simulink model "bh_2dof_RC_orientation"  (R2016a)
settings: Solver=VariableStepAuto  StartTime=0.0  StopTime=20  RelTol=1e-3
libraries: fl_lib x26, nesl_utility x10
settings Model: Creator=bhorton  LastModifiedBy=bhorton
settings DataIOCC: LimitDataPoints=on
settings DebuggingCC: AllowSymbolicDim=off
settings ModelReferenceCC: PropagateSignalLabelsOutOfModel=off
settings GRTTargetCC: GeneratePreprocessorConditionals=Use local settings

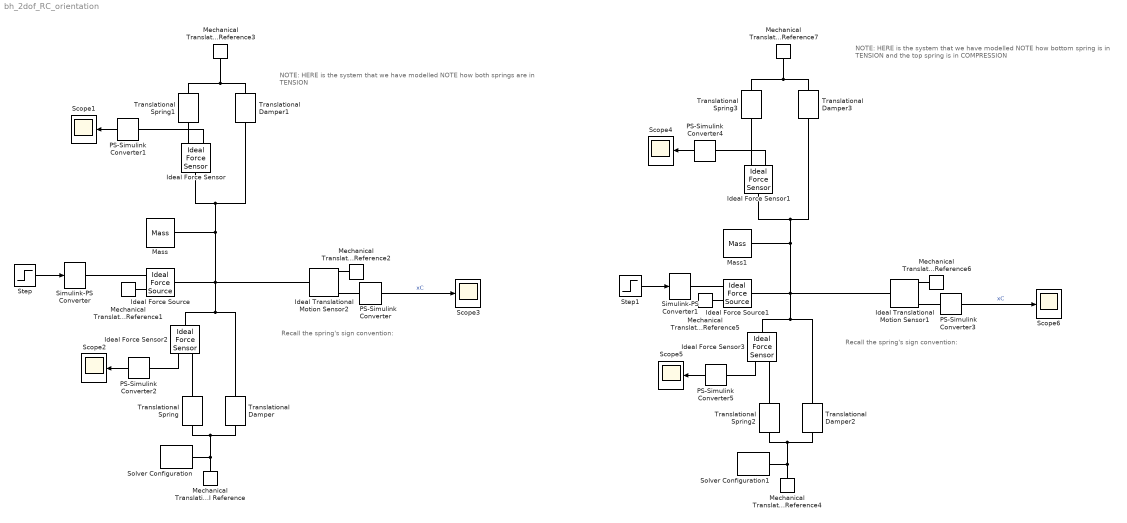
== system bh_2dof_RC_orientation ==
  note: NOTE:
      | HERE is the system that we have modelled
      | NOTE how both springs are in TENSION
  note: NOTE:
      | HERE is the system that we have modelled
      | NOTE how bottom spring is in TENSION and
      | the top spring is in COMPRESSION
  note: Recall the spring's sign convention:
  note: Recall the spring's sign convention:
  Ideal Force Sensor{,1..3} (4 alike) : fl_lib/Mechanical/Mechanical Sensors/Ideal Force Sensor
  Ideal Force Source : fl_lib/Mechanical/Mechanical Sources/Ideal Force Source
  Ideal Force Source1 : fl_lib/Mechanical/Mechanical Sources/Ideal Force Source
  Ideal Translational Motion Sensor1 : fl_lib/Mechanical/Mechanical Sensors/Ideal Translational Motion Sensor  offset=0 m
      settings: AttributesFormatString=OFFSET= %<offset>
  Ideal Translational Motion Sensor2 : fl_lib/Mechanical/Mechanical Sensors/Ideal Translational Motion Sensor  offset=0 m
      settings: AttributesFormatString=OFFSET= %<offset>
  Mass : fl_lib/Mechanical/Translational Elements/Mass  mass=1 kg  v_specify=off  v_priority=None  v=0 m/s  f_specify=off  f_priority=None  f=0 N
  Mass1 : fl_lib/Mechanical/Translational Elements/Mass  mass=1 kg  v_specify=off  v_priority=None  v=0 m/s  f_specify=off  f_priority=None  f=0 N
  Mechanical Translational Reference{,1..7} (8 alike) : fl_lib/Mechanical/Translational Elements/Mechanical Translational Reference
  PS-Simulink Converter : nesl_utility/PS-Simulink Converter  PhysicalDomain=network_engine_domain  SubClassName=ps_output  LeftPortType=input  RightPortType=output  PseudoPeriodic=off  Frequencies=[]  Unit=m  AffineConversion=off
  PS-Simulink Converter{1..2,4..5} (4 alike) : nesl_utility/PS-Simulink Converter  PhysicalDomain=network_engine_domain  SubClassName=ps_output  LeftPortType=input  RightPortType=output  PseudoPeriodic=off  Frequencies=[]  Unit=N  AffineConversion=off
  PS-Simulink Converter3 : nesl_utility/PS-Simulink Converter  PhysicalDomain=network_engine_domain  SubClassName=ps_output  LeftPortType=input  RightPortType=output  PseudoPeriodic=off  Frequencies=[]  Unit=m  AffineConversion=off
  Scope{1..6} (6 alike) : Scope
  Simulink-PS Converter : nesl_utility/Simulink-PS Converter  PhysicalDomain=network_engine_domain  SubClassName=ps_input  LeftPortType=input  RightPortType=output  PseudoPeriodic=off  Frequencies=[]  NoiseDistribution=none  NoiseParameters=[]  Unit=N  AffineConversion=off  InputFiltering=off  SimscapeFilterOrder=1  InputFilterTimeConstant=0.001  UdotUserProvided=1
  Simulink-PS Converter1 : nesl_utility/Simulink-PS Converter  PhysicalDomain=network_engine_domain  SubClassName=ps_input  LeftPortType=input  RightPortType=output  PseudoPeriodic=off  Frequencies=[]  NoiseDistribution=none  NoiseParameters=[]  Unit=N  AffineConversion=off  InputFiltering=off  SimscapeFilterOrder=1  InputFilterTimeConstant=0.001  UdotUserProvided=1
  Solver Configuration : nesl_utility/Solver Configuration  PhysicalDomain=network_engine_domain  SubClassName=solver  LeftPortType=input  RightPortType=generic  Accelerate=off  Tones=[]  Harmonics=[]  SimulateNoise=off  Profile=off  UseLocalSampling=off  EnableSwitchedLinearOptims=on  FrequencyDomain=off  UseCCode=off  RelTol=0.001  AbsTol=1e-06  MinStep=1e-09  ToWorkspace=off  RevertToSquareIcSolve=off  NumHomotopyIterations=100  PhasorMode=off  PhasorModeNumHarmonics=1  OverrideAbsTol=off  DoDC=off  ResidualTolerance=1e-09  UseLocalSolver=off  LocalSolverChoice=NE_BACKWARD_EULER_ADVANCER  LocalSolverSampleTime=0.001  DoFixedCost=off  MaxNonlinIter=3  MaxModeIter=2  LinearAlgebra=Sparse  DelaysMemoryBudget=1024  AutomaticFiltering=on  FilteringTimeConstant=0.001
  Solver Configuration1 : nesl_utility/Solver Configuration  PhysicalDomain=network_engine_domain  SubClassName=solver  LeftPortType=input  RightPortType=generic  Accelerate=off  Tones=[]  Harmonics=[]  SimulateNoise=off  Profile=off  UseLocalSampling=off  EnableSwitchedLinearOptims=on  FrequencyDomain=off  UseCCode=off  RelTol=0.001  AbsTol=1e-06  MinStep=1e-09  ToWorkspace=off  RevertToSquareIcSolve=off  NumHomotopyIterations=100  PhasorMode=off  PhasorModeNumHarmonics=1  OverrideAbsTol=off  DoDC=off  ResidualTolerance=1e-09  UseLocalSolver=off  LocalSolverChoice=NE_BACKWARD_EULER_ADVANCER  LocalSolverSampleTime=0.001  DoFixedCost=off  MaxNonlinIter=3  MaxModeIter=2  LinearAlgebra=Sparse  DelaysMemoryBudget=1024  AutomaticFiltering=on  FilteringTimeConstant=0.001
  Step : Step  Time=10  SampleTime=0
  Step1 : Step  Time=10  SampleTime=0
  Translational Damper{,1..3} (4 alike) : fl_lib/Mechanical/Translational Elements/Translational Damper  D=10 N/(m/s)  v_specify=off  v_priority=None  v=0 m/s  f_specify=off  f_priority=None  f=0 N
  Translational Spring{,1..3} (4 alike) : fl_lib/Mechanical/Translational Elements/Translational Spring  spr_rate=10 N/m  v_specify=off  v_priority=None  v=0 m/s  f_specify=off  f_priority=None  f=0 N  x_specify=off  x_priority=None  x=0 m
      settings: AttributesFormatString=K=%<spr_rate>
  wires:
  Step/1 -> Simulink-PS Converter/1
  PS-Simulink Converter/1 -> Scope3/1  "xC"
  PS-Simulink Converter2/1 -> Scope2/1
  PS-Simulink Converter1/1 -> Scope1/1
  Step1/1 -> Simulink-PS Converter1/1
  PS-Simulink Converter3/1 -> Scope6/1  "xC"
  PS-Simulink Converter5/1 -> Scope5/1
  PS-Simulink Converter4/1 -> Scope4/1
  connections:
  Translational Spring/LConn1 -- Mechanical Translational Reference/LConn1 -- Solver Configuration/RConn1 -- Translational Damper/LConn1
  Mechanical Translational Reference1/LConn1 -- Ideal Force Source/RConn2
  Simulink-PS Converter/RConn1 -- Ideal Force Source/RConn1
  Ideal Translational Motion Sensor2/RConn1 -- Mechanical Translational Reference2/LConn1
  Ideal Translational Motion Sensor2/RConn3 -- PS-Simulink Converter/LConn1
  Translational Damper1/RConn1 -- Mass/LConn1 -- Ideal Force Source/LConn1 -- Ideal Force Sensor2/LConn1 -- Translational Damper/RConn1 -- Ideal Translational Motion Sensor2/LConn1 -- Ideal Force Sensor/LConn1
  Translational Damper1/LConn1 -- Mechanical Translational Reference3/LConn1 -- Translational Spring1/LConn1
  Ideal Force Sensor/RConn1 -- Translational Spring1/RConn1
  Ideal Force Sensor2/RConn1 -- Translational Spring/RConn1
  PS-Simulink Converter2/LConn1 -- Ideal Force Sensor2/RConn2
  Ideal Force Sensor/RConn2 -- PS-Simulink Converter1/LConn1
  Translational Damper2/LConn1 -- Translational Spring2/LConn1 -- Mechanical Translational Reference4/LConn1 -- Solver Configuration1/RConn1
  Translational Damper3/LConn1 -- Ideal Force Sensor1/LConn1 -- Translational Damper2/RConn1 -- Ideal Force Sensor3/LConn1 -- Ideal Force Source1/LConn1 -- Ideal Translational Motion Sensor1/LConn1 -- Mass1/LConn1
  Ideal Force Sensor3/RConn1 -- Translational Spring2/RConn1
  Ideal Translational Motion Sensor1/RConn1 -- Mechanical Translational Reference6/LConn1
  PS-Simulink Converter5/LConn1 -- Ideal Force Sensor3/RConn2
  Simulink-PS Converter1/RConn1 -- Ideal Force Source1/RConn1
  Ideal Translational Motion Sensor1/RConn3 -- PS-Simulink Converter3/LConn1
  Mechanical Translational Reference5/LConn1 -- Ideal Force Source1/RConn2
  Translational Spring3/RConn1 -- Mechanical Translational Reference7/LConn1 -- Translational Damper3/RConn1
  Ideal Force Sensor1/RConn2 -- PS-Simulink Converter4/LConn1
  Translational Spring3/LConn1 -- Ideal Force Sensor1/RConn1
